simulink model "estimar_vThevenin"  (R2017b)
settings: Solver=ode8  StartTime=0.0  StopTime=time_sim  FixedStep=1/Fs  MaxStep=1e-4  RelTol=1e-3  EnableMultiTasking=on
values from neighbouring files (symbols this model uses):
  aT1 = V1t1/V2t1    (= 10.4545454545)    [prediccion.m]    (also in sensibilidad.m)
  aTeaf = V1eaf/V2eaf    (= 14.4736842105)    [prediccion.m]    (also in sensibilidad.m)
  f = 50    [hiperparametros.m]    (also in prediccion.m; sensibilidad.m)
  Fs = 4*Fm; save([PathFolder '/Fs'],'Fs')    [datos_entrenamiento.m]    (also in prediccion.m = 4*Fm; sensibilidad.m = 4*Fm)
  Leaf_pu = 0.1    [prediccion.m]    (also in sensibilidad.m)
  Lt1_pu = 0.12    [prediccion.m]    (also in sensibilidad.m)
  Reaf_pu = 0.01    [prediccion.m]    (also in sensibilidad.m)
  Rt1_pu = 0.012    [prediccion.m]    (also in sensibilidad.m)
  Rthe = 1.9    [prediccion.m]    (also in sensibilidad.m)
  Xthe = 5*37.7    (= 188.5)    [prediccion.m]    (also in sensibilidad.m)
  Zeaf_base_1 = V1eaf^2/(Seaf/3)    (= 12.1)    [prediccion.m]    (also in sensibilidad.m)
  Zsec = 1e-6    (= 1e-06)    [prediccion.m]    (also in sensibilidad.m)
  Zt1_base_1 = V1t1^2/(St1/3)    (= 944.642857143)    [prediccion.m]    (also in sensibilidad.m)
libraries: powerlib x1
PreSaveFcn:
  | RO=12.5;
  | L=3.6;
  | C1=0.000002;
  | C2=0.000020;
  | G=0.0005442;
  | 
  | I30=-1.810e-3;
  | V10=2.286;
  | V20=-222.014e-3;
  | 
  | E=1;
  | Ga=-757.576e-6;
  | Gb=-409.091e-6;
  | 
  | r0=10;
  | k1=3000;
  | k2=1.0;
  | k3=12.5;
  | 
  | m=0;
  | n=2;
settings Model: Creator=Administrador  LastModifiedBy=Jesser
settings DataIOCC: SaveFormat=Array  SignalLoggingSaveFormat=ModelDataLogs  TimeSaveName=t
settings OptimizationCC: ExpressionDepthLimit=2147483647  InitFltsAndDblsToZero=on  LifeSpan=inf
settings DebuggingCC: SaveWithParameterizedLinksMsg=none  UnderspecifiedInitializationDetection=Classic  MergeDetectMultiDrivingBlocksExec=none  SolverPrmCheckMsg=warning  FcnCallInpInsideContextMsg=warning  StateNameClashWarn=warning  StrictBusMsg=Warning  SFUnexpectedBacktrackingDiag=warning  SFNoUnconditionalDefaultTransitionDiag=warning  SFExecutionAtInitializationDiag=none
settings HardwareCC: ProdBitPerPointer=32  ProdBitPerSizeT=32  ProdBitPerPtrDiffT=32  ProdLargestAtomicFloat=None  ProdIntDivRoundTo=Undefined  ProdEndianess=Unspecified  ProdWordSize=32  ProdHWDeviceType=32-bit Generic
settings ModelReferenceCC: PropagateSignalLabelsOutOfModel=off
settings CodeAppCC: StateflowObjectComments=on
settings GRTTargetCC: TargetLangStandard=C89/C90 (ANSI)  CombineOutputUpdateFcns=off  GRTInterface=on
settings ConfigComp: CovMetricSettings=dw  CovHtmlReporting=on  CovSaveCumulativeToWorkspaceVar=on  CovSaveSingleToWorkspaceVar=on  CovExternalEMLEnable=off

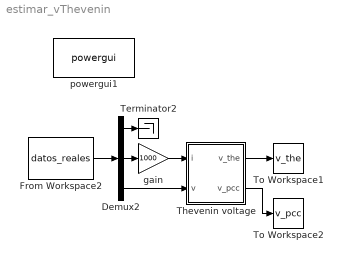
== system estimar_vThevenin ==
  Demux2 : Demux  Outputs=3
  From Workspace2 : FromWorkspace  VariableName=datos_reales  SampleTime=0
  Terminator2 : Terminator
  Thevenin voltage : Subsystem
  To Workspace1 : ToWorkspace  VariableName=v_the  SampleTime=-1
  To Workspace2 : ToWorkspace  VariableName=v_pcc  SampleTime=-1
  gain : Gain  Gain=1000
  powergui1 : powerlib/powergui  Priority=1  SimulationMode=Discrete  SampleTime=1/Fs  frequency=60  Iterations=50  frequencyindice=0  Pbase=100e6  ErrMax=1e-4  UnitsV=kV  UnitsW=MW  buscounter=0  FunctionMessages=off  echomessages=off  EnableUseOfTLC=off  CurrentSourceSwitches=off  DisableSnubberDevices=off  DisableRonSwitches=off  DisableVfSwitches=off  DisplayEquations=off  SolverType=Tustin/Backward Euler (TBE)  Interpol=off  ExternalGateDelay=off  methode=off  Ts=100  x0status=blocks  SPID=off  SwTol=0  HookPort=off  RestoreLinks=warning  ResistiveCurrentMeasurement=off  Frange=[0:2:500]  Ylog=off  Xlog=on  ShowGrid=off  save=off  variable=ZData  structure=0  ZoomFFT=off  StartTime=0.0  cycles=1  DisplayStyle=1  fundamental=60  FreqAxis=off  MaxFrequency=1000  frequencyindicesteady=1  RmsSteady=1  display=off
  wires:
  Thevenin voltage/1(v_the) -> To Workspace1/1
  From Workspace2/1 -> Demux2/1
  Demux2/1 -> Terminator2/1
  Demux2/3 -> Thevenin voltage/2(v)
  Demux2/2 -> gain/1
  gain/1 -> Thevenin voltage/1(i)
  Thevenin voltage/2(v_pcc) -> To Workspace2/1

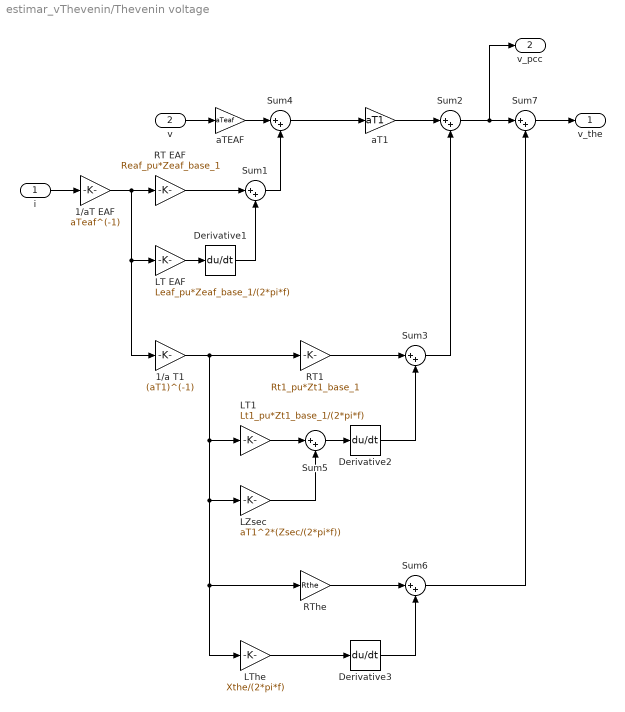
== system estimar_vThevenin/Thevenin voltage ==
  i : Inport
  v : Inport  Port=2
  1/a T1 : Gain  Gain=(aT1)^(-1)
  1/aT EAF : Gain  Gain=aTeaf^(-1)
  Derivative1 : Derivative
  Derivative2 : Derivative
  Derivative3 : Derivative
  LT EAF : Gain  Gain=Leaf_pu*Zeaf_base_1/(2*pi*f)
  LT1 : Gain  Gain=Lt1_pu*Zt1_base_1/(2*pi*f)
  LThe : Gain  Gain=Xthe/(2*pi*f)
  LZsec : Gain  Gain=aT1^2*(Zsec/(2*pi*f))
  RT EAF : Gain  Gain=Reaf_pu*Zeaf_base_1
  RT1 : Gain  Gain=Rt1_pu*Zt1_base_1
  RThe : Gain  Gain=Rthe
  Sum{1..7} (7 alike) : Sum  Inputs=|++
  aT1 : Gain  Gain=aT1
  aTEAF : Gain  Gain=aTeaf
  v_the : Outport
  v_pcc : Outport  Port=2
  wires:
  Sum7/1 -> v_the/1
  Sum6/1 -> Sum7/2
  Sum2/1 -> v_pcc/1, Sum7/1
  Derivative3/1 -> Sum6/2
  RThe/1 -> Sum6/1
  Derivative2/1 -> Sum3/2
  RT1/1 -> Sum3/1
  aT1/1 -> Sum2/1
  Derivative1/1 -> Sum1/2
  Sum1/1 -> Sum4/2
  RT EAF/1 -> Sum1/1
  1/aT EAF/1 -> RT EAF/1, 1/a T1/1, LT EAF/1
  aTEAF/1 -> Sum4/1
  Sum4/1 -> aT1/1
  Sum5/1 -> Derivative2/1
  LT EAF/1 -> Derivative1/1
  LZsec/1 -> Sum5/2
  i/1 -> 1/aT EAF/1
  1/a T1/1 -> LT1/1, LThe/1, RThe/1, LZsec/1, RT1/1
  LThe/1 -> Derivative3/1
  LT1/1 -> Sum5/1
  v/1 -> aTEAF/1
  Sum3/1 -> Sum2/2
